simulink library "UBCSailbotBlocks"  (R2020a)
settings: Solver=VariableStepAuto  StartTime=0.0  StopTime=10.0  RelTol=1e-3
libraries: simulink x1, $bdroot x1
settings Model: Creator=bruce  LastModifiedBy=bruce

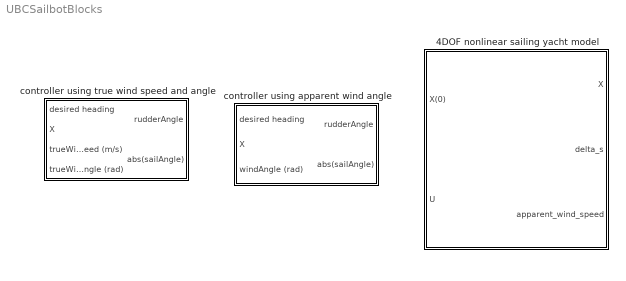
== system UBCSailbotBlocks ==
  4DOF nonlinear sailing yacht model : Subsystem
  controller using apparent wind angle : Subsystem  AncestorBlock=UBCSailbotBlocks/controller
  controller using true wind speed and angle : Subsystem

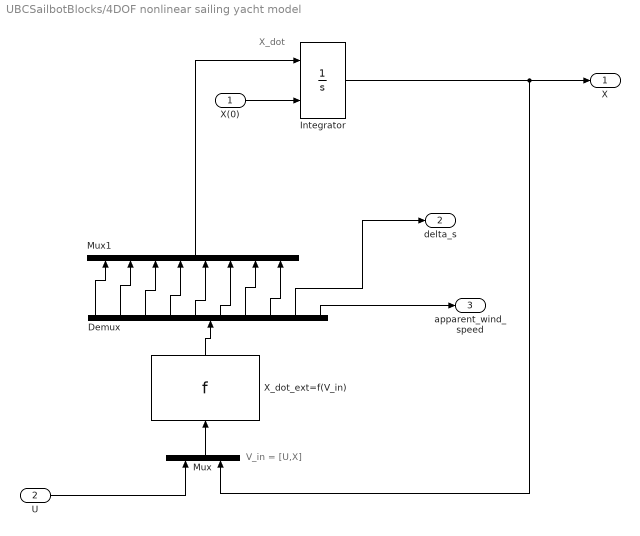
== system UBCSailbotBlocks/4DOF nonlinear sailing yacht model ==
  note: V_in = [U,X]
  note: X_dot
  X(0) : Inport
  U : Inport  Port=2
  Demux : Demux  Outputs=10
  Integrator : Integrator  InitialConditionSource=external  InitialCondition=[0;0;0;pi;1;0;0;0]
  Mux : Mux  Inputs=2
  Mux1 : Mux  Inputs=8
  X_dot_ext=f(V_in) : MATLABFcn  MATLABFcn=f  OutputDimensions=10
  X : Outport
  delta_s : Outport  Port=2
  apparent_wind_speed : Outport  Port=3
  wires:
  Mux1/1 -> Integrator/1
  Demux/1 -> Mux1/1
  Demux/2 -> Mux1/2
  Demux/3 -> Mux1/3
  Demux/4 -> Mux1/4
  Demux/5 -> Mux1/5
  Demux/6 -> Mux1/6
  Demux/7 -> Mux1/7
  Demux/8 -> Mux1/8
  Demux/9 -> delta_s/1
  X_dot_ext=f(V_in)/1 -> Demux/1
  Integrator/1 -> Mux/2, X/1
  U/1 -> Mux/1
  Mux/1 -> X_dot_ext=f(V_in)/1
  X(0)/1 -> Integrator/2
  Demux/10 -> apparent_wind_speed/1

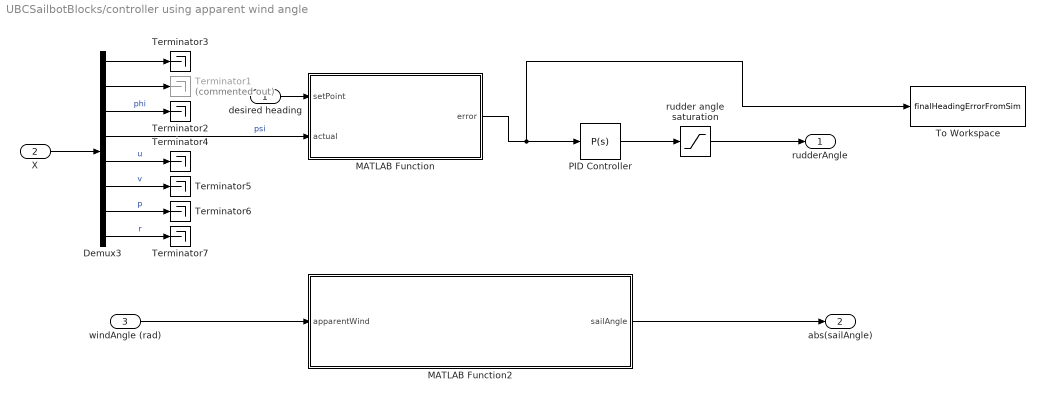
== system UBCSailbotBlocks/controller using apparent wind angle ==
  desired heading : Inport
  X : Inport  Port=2
  windAngle (rad) : Inport  Port=3
  Demux3 : Demux  Outputs=8
  MATLAB Function : MATLAB Function  TreatAsAtomicUnit=on
  MATLAB Function2 : MATLAB Function  TreatAsAtomicUnit=on
  PID Controller : simulink/Continuous/PID Controller  Controller=P  Form=Parallel  TimeDomain=Continuous-time  UseExternalTs=off  SampleTime=-1  IntegratorMethod=Forward Euler  FilterMethod=Forward Euler  ControllerParametersSource=internal  P=0.5  I=0  D=0  UseFilter=on  N=100  TunerSelectOption=Transfer Function Based (PID Tuner App)  InitialConditionSource=internal  InitialConditionForIntegrator=0  InitialConditionForFilter=0  DifferentiatorICPrevScaledInput=0  ExternalReset=none  TrackingMode=off  Kt=1  LimitOutput=off  UpperSaturationLimit=inf  LowerSaturationLimit=-inf  LinearizeAsGain=on  AntiWindupMode=none  Kb=1  POutMin=[]  POutMax=[]  IOutMin=[]  IOutMax=[]  DOutMin=[]  DOutMax=[]  NOutMin=[]  NOutMax=[]  SumOutMin=[]  SumOutMax=[]  SaturationOutMin=[]  SaturationOutMax=[]  PParamMin=[]  PParamMax=[]  IParamMin=[]  IParamMax=[]  DParamMin=[]  DParamMax=[]  NParamMin=[]  NParamMax=[]  KbParamMin=[]  KbParamMax=[]  KtParamMin=[]  KtParamMax=[]  KbOutMin=[]  KbOutMax=[]  KtOutMin=[]  KtOutMax=[]  IntegratorOutMin=[]  IntegratorOutMax=[]  FilterOutMin=[]  FilterOutMax=[]  SumI1OutMin=[]  SumI1OutMax=[]  SumI2OutMin=[]  SumI2OutMax=[]  SumI3OutMin=[]  SumI3OutMax=[]  SumI4OutMin=[]  SumI4OutMax=[]  SumDOutMin=[]  SumDOutMax=[]  DifferentiatorOutMin=[]  DifferentiatorOutMax=[]  FilterDiffOutCoefMin=[]  FilterDiffOutCoefMax=[]  ReciprocalOutMin=[]  ReciprocalOutMax=[]  SumDenOutMin=[]  SumDenOutMax=[]  SumNumOutMin=[]  SumNumOutMax=[]  DivideOutMin=[]  DivideOutMax=[]  UdiffTsProdOutMin=[]  UdiffTsProdOutMax=[]  NTsProdOutMin=[]  NTsProdOutMax=[]  UintegralTsProdOutMin=[]  UintegralTsProdOutMax=[]  UngainTsProdOutMin=[]  UngainTsProdOutMax=[]  IntegratorContinuousStateAttributes=''  IntegratorStateMustResolveToSignalObject=off  IntegratorRTWStateStorageClass=Auto  FilterContinuousStateAttributes=''  FilterStateMustResolveToSignalObject=off  FilterRTWStateStorageClass=Auto  ParallelPVariant=InternalParameters  IdealPVariant=Disabled  IVariant=Disabled  DVariant=Disabled  IntegratorVariant=Disabled  SatVariant=Disabled  AWVariant=Disabled  PCopyVariant=Disabled  TRVariant=Disabled  FdbkBlocksVariant=Forward  IdealPFdbkVariant=Disabled  SatFdbkVariant=Disabled  DerivativeFilterVariant=Disabled  NVariant=Disabled  NCopyVariant=Disabled_SignalSpec  FilterICVariant=Disabled  IntegratorICVariant=Disabled  ExternalResetVariant=Disabled  TRSumVariant=Passthrough  SumFdbkVariant=Disabled  SumVariant=Passthrough_P  TsampFilterVariant=InternalTs  TsampNgainVariant=Passthrough  TsampIntegralVariant=Disabled_SignalSpec
  Terminator1 : Terminator  Commented=on
  Terminator{2..7} (6 alike) : Terminator
  To Workspace : ToWorkspace  VariableName=finalHeadingErrorFromSim  SampleTime=-1
      settings: MaxDataPoints=1  Save2DSignal=2-D array (concatenate along first dimension)
  rudder angle saturation : Saturate  UpperLimit=pi/3  LowerLimit=-pi/3  LinearizeAsGain=off
  rudderAngle : Outport
  abs(sailAngle) : Outport  Port=2
  wires:
  Demux3/4 -> MATLAB Function/2(actual)  "psi"
  X/1 -> Demux3/1
  Demux3/1 -> Terminator3/1
  Demux3/2 -> Terminator1/1
  Demux3/3 -> Terminator2/1  "phi"
  Demux3/5 -> Terminator4/1  "u"
  Demux3/6 -> Terminator5/1  "v"
  Demux3/7 -> Terminator6/1  "p"
  Demux3/8 -> Terminator7/1  "r"
  desired heading/1 -> MATLAB Function/1(setPoint)
  rudder angle saturation/1 -> rudderAngle/1
  MATLAB Function/1(error) -> To Workspace/1, PID Controller/1
  PID Controller/1 -> rudder angle saturation/1
  windAngle (rad)/1 -> MATLAB Function2/1(apparentWind)
  MATLAB Function2/1(sailAngle) -> abs(sailAngle)/1

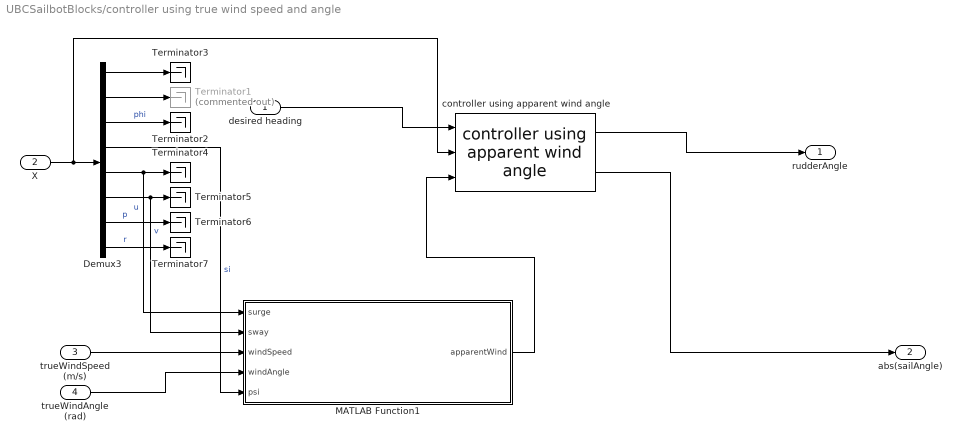
== system UBCSailbotBlocks/controller using true wind speed and angle ==
  desired heading : Inport
  X : Inport  Port=2
  trueWindSpeed (m/s) : Inport  Port=3
  trueWindAngle (rad) : Inport  Port=4
  Demux3 : Demux  Outputs=8
  MATLAB Function1 : MATLAB Function  TreatAsAtomicUnit=on
  Terminator1 : Terminator  Commented=on
  Terminator{2..7} (6 alike) : Terminator
  controller using apparent wind angle : $bdroot/controller using apparent wind angle  SystemSampleTime=-1  Latency=0  AutoFrameSizeCalculation=off
  rudderAngle : Outport
  abs(sailAngle) : Outport  Port=2
  wires:
  Demux3/4 -> MATLAB Function1/5(psi)  "si"
  X/1 -> controller using apparent wind angle/2, Demux3/1
  Demux3/1 -> Terminator3/1
  Demux3/2 -> Terminator1/1
  Demux3/3 -> Terminator2/1  "phi"
  Demux3/5 -> MATLAB Function1/1(surge), Terminator4/1  "u"
  Demux3/6 -> MATLAB Function1/2(sway), Terminator5/1  "v"
  Demux3/7 -> Terminator6/1  "p"
  Demux3/8 -> Terminator7/1  "r"
  desired heading/1 -> controller using apparent wind angle/1
  trueWindSpeed (m/s)/1 -> MATLAB Function1/3(windSpeed)
  trueWindAngle (rad)/1 -> MATLAB Function1/4(windAngle)
  MATLAB Function1/1(apparentWind) -> controller using apparent wind angle/3
  controller using apparent wind angle/2 -> abs(sailAngle)/1
  controller using apparent wind angle/1 -> rudderAngle/1

== matlab function UBCSailbotBlocks/controller using true wind speed and angle/MATLAB Function1 ==
  data: surge input; apparentWind output; sway input; windSpeed input; windAngle input; psi input
function apparentWind = getApparentWindAngleWrapper(surge, sway, windSpeed, windAngle, psi)

apparentWind = getApparentWindAngle(surge, sway, windSpeed, windAngle, psi);

== matlab function UBCSailbotBlocks/controller using apparent wind angle/MATLAB Function ==
  data: setPoint input; error output; actual input
function error = getHeadingError(setPoint,actual)
error = getHeadingError(setPoint,actual);
end

== matlab function UBCSailbotBlocks/controller using apparent wind angle/MATLAB Function2 ==
  data: apparentWind input; sailAngle output
function sailAngle = getSailAngleWrapper(apparentWind)

sailAngle = getSailAngle(apparentWind);
